simulink model "LQR_Reference_Tracking_Constant_Vx_Cf_Cr_Sim"  (R2018a)
settings: Solver=FixedStepDiscrete  StartTime=0.0  StopTime=t_final  FixedStep=T  RelTol=1e-3
values from neighbouring files (symbols this model uses):
  Ad = sysd.a    [LQR_Ref_Track_Const_Vx_Cf_Cr_LinMod_3_state.m]
  Bd = sysd.b    [LQR_Ref_Track_Const_Vx_Cf_Cr_LinMod_3_state.m]
  K_lqr = Kd(1:3)    [LQR_Ref_Track_Const_Vx_Cf_Cr_LinMod_3_state.m]
  Ki = Kd(4)    [LQR_Ref_Track_Const_Vx_Cf_Cr_LinMod_3_state.m]
undefined symbols (not defined in the file or in its folder): DiscIntNeverNeededParam, Kd
settings Model: Creator=Shouvik Chakraborty  LastModifiedBy=Shouvik Chakraborty

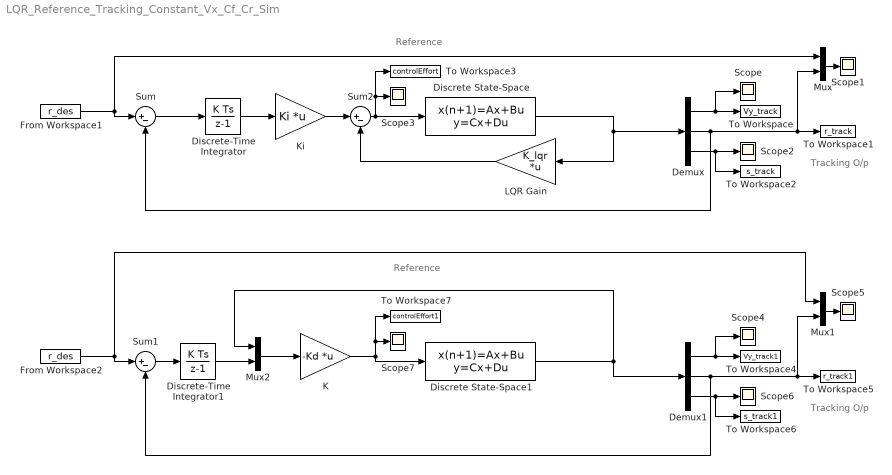
== system LQR_Reference_Tracking_Constant_Vx_Cf_Cr_Sim ==
  note: Reference
  note: Tracking O/p
  note: Reference
  note: Tracking O/p
  Demux : Demux  Outputs=3
  Demux1 : Demux  Outputs=3
  Discrete State-Space : DiscreteStateSpace  A=Ad  B=Bd  C=eye(3,3)  D=[0;0;0]  SampleTime=-1
  Discrete State-Space1 : DiscreteStateSpace  A=Ad  B=Bd  C=eye(3,3)  D=[0;0;0]  SampleTime=-1
  Discrete-Time Integrator : DiscreteIntegrator  SampleTime=-1  ICPrevOutput=DiscIntNeverNeededParam  ICPrevScaledInput=DiscIntNeverNeededParam
  Discrete-Time Integrator1 : DiscreteIntegrator  SampleTime=-1  ICPrevOutput=DiscIntNeverNeededParam  ICPrevScaledInput=DiscIntNeverNeededParam
  From Workspace1 : FromWorkspace  VariableName=r_des  SampleTime=0
  From Workspace2 : FromWorkspace  VariableName=r_des  SampleTime=0
  K : Gain  Gain=-Kd  Multiplication=Matrix(K*u)
  Ki : Gain  Gain=Ki  Multiplication=Matrix(K*u)
  LQR Gain : Gain  Gain=K_lqr  Multiplication=Matrix(K*u)
  Mux : Mux  Inputs=2
  Mux1 : Mux  Inputs=2
  Mux2 : Mux  Inputs=2
  Scope{,1..7} (8 alike) : Scope
  Sum : Sum  Inputs=|+-
  Sum1 : Sum  Inputs=|+-
  Sum2 : Sum  Inputs=|+-
  To Workspace : ToWorkspace  VariableName=Vy_track  SampleTime=-1
  To Workspace1 : ToWorkspace  VariableName=r_track  SampleTime=-1
  To Workspace2 : ToWorkspace  VariableName=s_track  SampleTime=-1
  To Workspace3 : ToWorkspace  VariableName=controlEffort  SampleTime=-1
  To Workspace4 : ToWorkspace  VariableName=Vy_track1  SampleTime=-1
  To Workspace5 : ToWorkspace  VariableName=r_track1  SampleTime=-1
  To Workspace6 : ToWorkspace  VariableName=s_track1  SampleTime=-1
  To Workspace7 : ToWorkspace  VariableName=controlEffort1  SampleTime=-1
  wires:
  Demux/1 -> Scope/1, To Workspace/1
  Sum/1 -> Discrete-Time Integrator/1
  Discrete-Time Integrator/1 -> Ki/1
  Sum2/1 -> To Workspace3/1, Scope3/1, Discrete State-Space/1
  Discrete State-Space/1 -> Demux/1, LQR Gain/1
  LQR Gain/1 -> Sum2/2
  From Workspace1/1 -> Sum/1, Mux/1
  Ki/1 -> Sum2/1
  Demux/2 -> Sum/2, Mux/2, To Workspace1/1
  Demux/3 -> To Workspace2/1, Scope2/1
  Mux/1 -> Scope1/1
  Mux1/1 -> Scope5/1
  Demux1/1 -> Scope4/1, To Workspace4/1
  Demux1/2 -> Sum1/2, Mux1/2, To Workspace5/1
  Demux1/3 -> To Workspace6/1, Scope6/1
  Discrete State-Space1/1 -> Demux1/1, Mux2/1
  From Workspace2/1 -> Sum1/1, Mux1/1
  K/1 -> Discrete State-Space1/1, To Workspace7/1, Scope7/1
  Sum1/1 -> Discrete-Time Integrator1/1
  Discrete-Time Integrator1/1 -> Mux2/2
  Mux2/1 -> K/1
